simulink model "yarpRemotePosEnc"  (Simulink 7.3)
settings: Solver=ode45  SolverMode=SingleTasking  StartTime=0.0  StopTime=inf  RelTol=1e-3  AbsTol=1e-6
libraries: utility x1
settings Model: Creator=dmedonza  LastModifiedBy=yo
settings DataIOCC: SaveOutput=off  SignalLogging=off  SaveTime=off
settings OptimizationCC: BooleanDataType=off
settings DebuggingCC: SaveWithParameterizedLinksMsg=none  SignalResolutionControl=TryResolveAllWithWarning  SolverPrmCheckMsg=none  MultiTaskDSMMsg=warning  MultiTaskCondExecSysMsg=none  StrictBusMsg=None
settings HardwareCC: TargetUnknown=on
settings RTWCC: TemplateMakefile=grt_vc.tmf  IncludeERTFirstTime=on

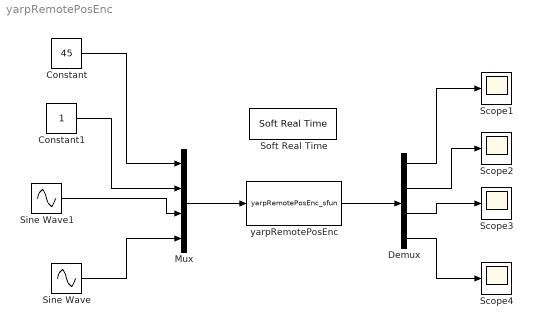
== system yarpRemotePosEnc ==
  Constant : Constant  Value=45  OutDataType=fixdt(1, 16)  OutScaling=2^0
  Constant1 : Constant  OutDataType=fixdt(1, 16)  OutScaling=2^0
  Demux : Demux
  Mux : Mux
  Scope{1..4} (4 alike) : Scope
      Scope1 settings: TimeRange=10  YMin=0  YMax=45
      Scope2 settings: YMin=0  YMax=1
      Scope3 settings: TimeRange=10  YMin=-100  YMax=75  SaveName=ScopeData2
      Scope4 settings: YMin=-100  YMax=100  SaveName=ScopeData3
  Sine Wave : Sin  Amplitude=90  Bias=0  Frequency=0.5  Phase=0  Samples=10  SampleTime=0  Offset=0
  Sine Wave1 : Sin  Amplitude=90  Bias=0  Frequency=0.5  Phase=pi  Samples=10  SampleTime=0  Offset=0
  Soft Real Time : utility/Soft Real Time  x=1
  yarpRemotePosEnc : S-Function  FunctionName=yarpRemotePosEnc_sfun  Parameters='/controlboard' 4  EnableBusSupport=off
      mask Display: image(imread('yarpPipes.png'))
  wires:
  Demux/1 -> Scope1/1
  Demux/2 -> Scope2/1
  Demux/3 -> Scope3/1
  Demux/4 -> Scope4/1
  yarpRemotePosEnc/1 -> Demux/1
  Mux/1 -> yarpRemotePosEnc/1
  Constant/1 -> Mux/1
  Constant1/1 -> Mux/2
  Sine Wave/1 -> Mux/4
  Sine Wave1/1 -> Mux/3
